simulink model "PMSM_Drive_ForFlight"  (R2025a)
settings: Solver=ode4  StartTime=0.0  StopTime=StopTime  FixedStep=Ts_solver  RelTol=1e-3
values from neighbouring files (symbols this model uses):
  Bm = 1e-3    (= 0.001)    [EMRAX348_DQData.m]    (also in Evolito_D500_DQData.m; pmsm_batt_testbench_data.m)
  C1_pack = (Np/Ns)*c1_cell    [pmsm_batt_testbench_data.m]
  Cap_pack = Np*Cell_Cap    (= 220.5)    [pmsm_batt_testbench_data.m]
  Imax = 1070    [EMRAX348_DQData.m]    (also in Evolito_D500_DQData.m = 1450; pmsm_batt_testbench_data.m = 800)
  Jm_flight = 0.09    [pmsm_batt_testbench_data.m]
  Ki_i = Rs*bw_i    (= 62.8318530718)    [pmsm_batt_testbench_data.m]
  Kp_i = Ld*bw_i    (= 1.25663706144)    [pmsm_batt_testbench_data.m]
  Kt = 1.5*p*psim    (= 3.6)    [pmsm_batt_testbench_data.m]
  Ld = 52e-6    (= 5.2e-05)    [EMRAX348_DQData.m]    (also in Evolito_D500_DQData.m = 4e-05; pmsm_batt_testbench_data.m = 0.0002)
  Lq = 52e-6    (= 5.2e-05)    [EMRAX348_DQData.m]    (also in Evolito_D500_DQData.m = 4e-05; pmsm_batt_testbench_data.m = 0.0002)
  OCV_pack = Ns*ocv_cell    [pmsm_batt_testbench_data.m]
  p = 10    [EMRAX348_DQData.m]    (also in Evolito_D500_DQData.m; pmsm_batt_testbench_data.m = 15)
  psim = 0.06249    [EMRAX348_DQData.m]    (also in Evolito_D500_DQData.m = 0.045; pmsm_batt_testbench_data.m = 0.16)
  R0_pack = (Ns/Np)*rs_cell    [pmsm_batt_testbench_data.m]
  R1_pack = (Ns/Np)*r1_cell    [pmsm_batt_testbench_data.m]
  Rs = 0.00474    [EMRAX348_DQData.m]    (also in Evolito_D500_DQData.m = 0.004; pmsm_batt_testbench_data.m = 0.01)
  SOC0 = 0.90    (= 0.9)    [pmsm_batt_testbench_data.m]
  tau_dc = 1e-4    (= 0.0001)    [pmsm_batt_testbench_data.m]
  trqR_hover = [1500; 1505; 1500; 1505]    [pmsm_batt_testbench_data.m]
undefined symbols (not defined in the file or in its folder): soc_bp
libraries: slpidlib x2, simulink x1
settings Model: Creator=froshoo  LastModifiedBy=wu2408

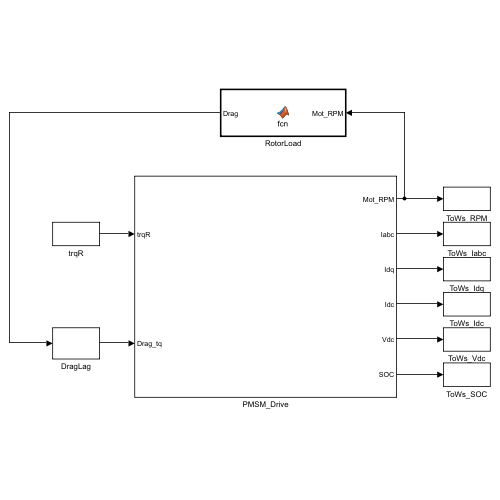
[thumbnail: Simulink's stored preview of the top-level diagram]
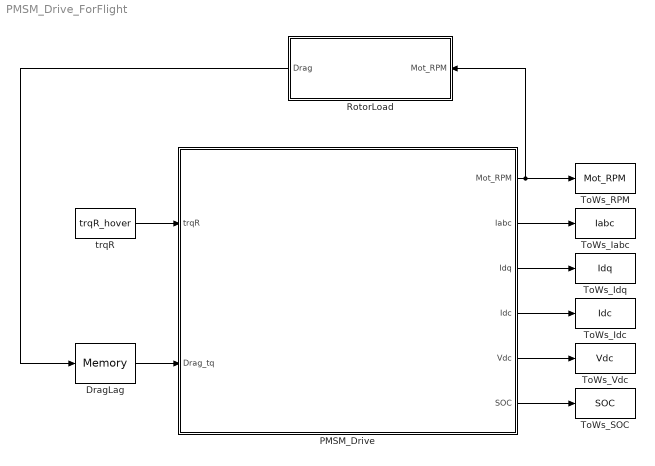
== system PMSM_Drive_ForFlight ==
  DragLag : Memory
  PMSM_Drive : Subsystem
  RotorLoad : MATLAB Function  TreatAsAtomicUnit=on
  ToWs_Iabc : ToWorkspace  VariableName=Iabc  SaveFormat=Timeseries  SampleTime=-1
  ToWs_Idc : ToWorkspace  VariableName=Idc  SaveFormat=Timeseries  SampleTime=-1
  ToWs_Idq : ToWorkspace  VariableName=Idq  SaveFormat=Timeseries  SampleTime=-1
  ToWs_RPM : ToWorkspace  VariableName=Mot_RPM  SaveFormat=Timeseries  SampleTime=-1
  ToWs_SOC : ToWorkspace  VariableName=SOC  SaveFormat=Timeseries  SampleTime=-1
  ToWs_Vdc : ToWorkspace  VariableName=Vdc  SaveFormat=Timeseries  SampleTime=-1
  trqR : Constant  Value=trqR_hover
  wires:
  trqR/1 -> PMSM_Drive/1(trqR)
  RotorLoad/1(Drag) -> DragLag/1
  DragLag/1 -> PMSM_Drive/2(Drag_tq)
  PMSM_Drive/1(Mot_RPM) -> RotorLoad/1(Mot_RPM), ToWs_RPM/1
  PMSM_Drive/2(Iabc) -> ToWs_Iabc/1
  PMSM_Drive/3(Idq) -> ToWs_Idq/1
  PMSM_Drive/4(Idc) -> ToWs_Idc/1
  PMSM_Drive/5(Vdc) -> ToWs_Vdc/1
  PMSM_Drive/6(SOC) -> ToWs_SOC/1

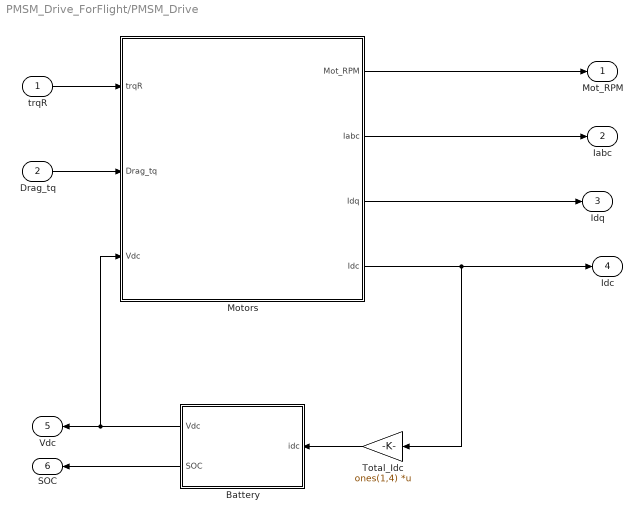
== system PMSM_Drive_ForFlight/PMSM_Drive ==
  trqR : Inport
  Drag_tq : Inport  Port=2
  Battery : Subsystem
  Motors : Subsystem  TreatAsAtomicUnit=on
  Total_Idc : Gain  Gain=ones(1,4)  Multiplication=Matrix(K*u)
  Mot_RPM : Outport
  Iabc : Outport  Port=2
  Idq : Outport  Port=3
  Idc : Outport  Port=4
  Vdc : Outport  Port=5
  SOC : Outport  Port=6
  wires:
  trqR/1 -> Motors/1(trqR)
  Drag_tq/1 -> Motors/2(Drag_tq)
  Battery/1(Vdc) -> Vdc/1, Motors/3(Vdc)
  Motors/1(Mot_RPM) -> Mot_RPM/1
  Motors/2(Iabc) -> Iabc/1
  Motors/3(Idq) -> Idq/1
  Motors/4(Idc) -> Total_Idc/1, Idc/1
  Total_Idc/1 -> Battery/1(idc)
  Battery/2(SOC) -> SOC/1

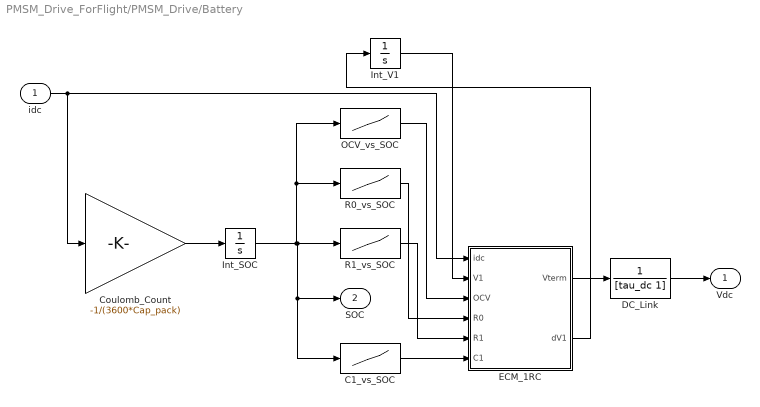
== system PMSM_Drive_ForFlight/PMSM_Drive/Battery ==
  idc : Inport
  C1_vs_SOC : Lookup_n-D  NumberOfTableDimensions=1  BreakpointsForDimension1=soc_bp  Table=C1_pack  InternalRulePriority=Speed  RndMeth=Simplest
  Coulomb_Count : Gain  Gain=-1/(3600*Cap_pack)
  DC_Link : TransferFcn  Denominator=[tau_dc 1]
  ECM_1RC : MATLAB Function  TreatAsAtomicUnit=on
  Int_SOC : Integrator  InitialCondition=SOC0
  Int_V1 : Integrator
  OCV_vs_SOC : Lookup_n-D  NumberOfTableDimensions=1  BreakpointsForDimension1=soc_bp  Table=OCV_pack  InternalRulePriority=Speed  RndMeth=Simplest
  R0_vs_SOC : Lookup_n-D  NumberOfTableDimensions=1  BreakpointsForDimension1=soc_bp  Table=R0_pack  InternalRulePriority=Speed  RndMeth=Simplest
  R1_vs_SOC : Lookup_n-D  NumberOfTableDimensions=1  BreakpointsForDimension1=soc_bp  Table=R1_pack  InternalRulePriority=Speed  RndMeth=Simplest
  Vdc : Outport
  SOC : Outport  Port=2
  wires:
  Int_V1/1 -> ECM_1RC/2(V1)
  idc/1 -> ECM_1RC/1(idc), Coulomb_Count/1
  Coulomb_Count/1 -> Int_SOC/1
  R0_vs_SOC/1 -> ECM_1RC/4(R0)
  Int_SOC/1 -> C1_vs_SOC/1, SOC/1, R1_vs_SOC/1, OCV_vs_SOC/1, R0_vs_SOC/1
  OCV_vs_SOC/1 -> ECM_1RC/3(OCV)
  R1_vs_SOC/1 -> ECM_1RC/5(R1)
  C1_vs_SOC/1 -> ECM_1RC/6(C1)
  ECM_1RC/1(Vterm) -> DC_Link/1
  ECM_1RC/2(dV1) -> Int_V1/1
  DC_Link/1 -> Vdc/1

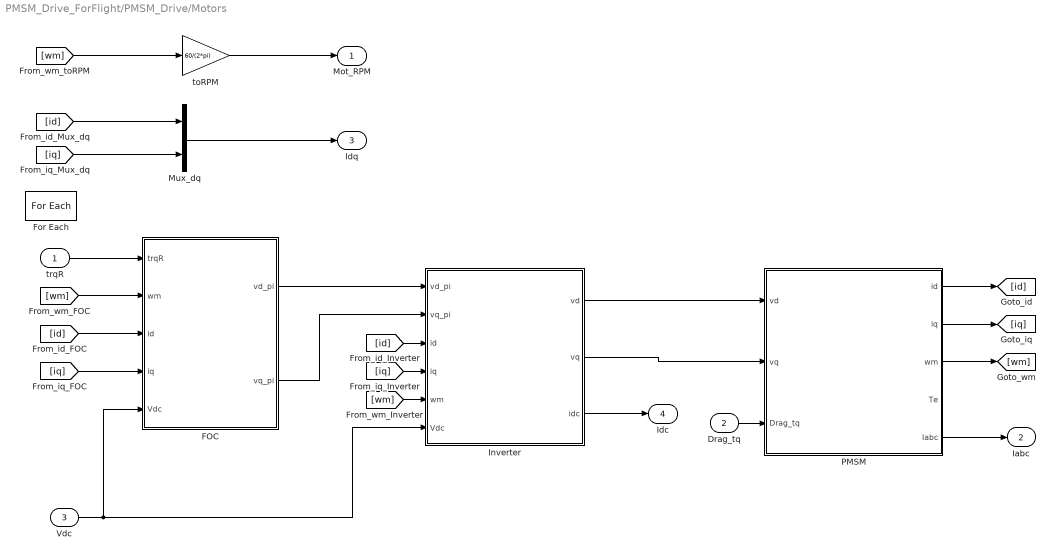
== system PMSM_Drive_ForFlight/PMSM_Drive/Motors ==
  trqR : Inport  Partition=on  PartitionDimension=1  PartitionWidth=1  PartitionOffset=0
  Drag_tq : Inport  Port=2  Partition=on  PartitionDimension=1  PartitionWidth=1  PartitionOffset=0
  Vdc : Inport  Port=3
  FOC : Subsystem
  For Each : ForEach  DisableCoverage=on  SpecifiedNumIters=4
  Inverter : Subsystem
  Mux_dq : Mux  Inputs=2
  PMSM : Subsystem
  toRPM : Gain  Gain=60/(2*pi)
  Mot_RPM : Outport  ConcatenationDimension=1
  Iabc : Outport  Port=2  ConcatenationDimension=1
  Idq : Outport  Port=3  ConcatenationDimension=1
  Idc : Outport  Port=4  ConcatenationDimension=1
  wires:
  [wm] -> Inverter/5(wm)
  [wm] -> toRPM/1
  [iq] -> Mux_dq/2
  [wm] -> FOC/2(wm)
  PMSM/5(Iabc) -> Iabc/1
  PMSM/3(wm) -> [wm]
  [id] -> Mux_dq/1
  trqR/1 -> FOC/1(trqR)
  [id] -> FOC/3(id)
  [iq] -> Inverter/4(iq)
  [iq] -> FOC/4(iq)
  Vdc/1 -> Inverter/6(Vdc), FOC/5(Vdc)
  toRPM/1 -> Mot_RPM/1
  Mux_dq/1 -> Idq/1
  FOC/2(vq_pi) -> Inverter/2(vq_pi)
  FOC/1(vd_pi) -> Inverter/1(vd_pi)
  [id] -> Inverter/3(id)
  Inverter/3(idc) -> Idc/1
  Inverter/2(vq) -> PMSM/2(vq)
  Inverter/1(vd) -> PMSM/1(vd)
  Drag_tq/1 -> PMSM/3(Drag_tq)
  PMSM/2(iq) -> [iq]
  PMSM/1(id) -> [id]

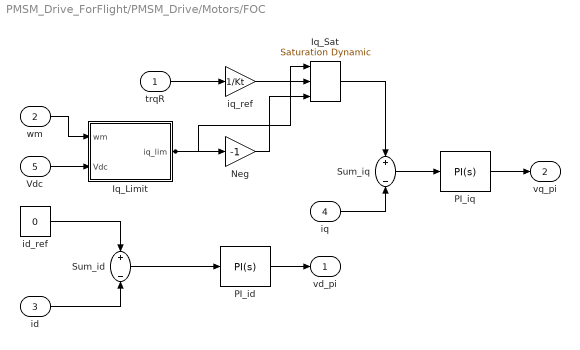
== system PMSM_Drive_ForFlight/PMSM_Drive/Motors/FOC ==
  trqR : Inport
  wm : Inport  Port=2
  id : Inport  Port=3
  iq : Inport  Port=4
  Vdc : Inport  Port=5
  Iq_Limit : MATLAB Function  TreatAsAtomicUnit=on
  Iq_Sat : simulink/Discontinuities/Saturation Dynamic  OutMin=[]  OutMax=[]  OutDataTypeStr=Inherit: Same as second input  OutDataType=fixdt(1, 16)  OutScaling=2^-10  DoSatur=off
  Neg : Gain  Gain=-1
  PI_id : slpidlib/PID Controller  Controller=PI  Form=Parallel  TimeDomain=Continuous-time  UseExternalTs=off  SampleTime=-1  IntegratorMethod=Forward Euler  FilterMethod=Forward Euler  ControllerParametersSource=internal  P=Kp_i  I=Ki_i  UseKiTs=off  D=0  UseExternalDerivativeSource=off  N=100  UseFilter=on  TunerSelectOption=Transfer Function Based (PID Tuner App)  InitialConditionSource=internal  InitialConditionForIntegrator=0  InitialConditionForFilter=0  DifferentiatorICPrevScaledInput=0  ExternalReset=none  TrackingMode=off  Kt=1  LimitOutput=off  SatLimitsSource=internal  UpperSaturationLimit=inf  LowerSaturationLimit=-inf  LinearizeAsGain=on  AntiWindupMode=none  Kb=1  LimitIntegrator=off  UpperIntegratorSaturationLimit=inf  LowerIntegratorSaturationLimit=-inf  POutMin=[]  POutMax=[]  IOutMin=[]  IOutMax=[]  DOutMin=[]  DOutMax=[]  NOutMin=[]  NOutMax=[]  SumOutMin=[]  SumOutMax=[]  SaturationOutMin=[]  SaturationOutMax=[]  PParamMin=[]  PParamMax=[]  IParamMin=[]  IParamMax=[]  DParamMin=[]  DParamMax=[]  NParamMin=[]  NParamMax=[]  KbParamMin=[]  KbParamMax=[]  KtParamMin=[]  KtParamMax=[]  KbOutMin=[]  KbOutMax=[]  KtOutMin=[]  KtOutMax=[]  IntegratorOutMin=[]  IntegratorOutMax=[]  FilterOutMin=[]  FilterOutMax=[]  SumI1OutMin=[]  SumI1OutMax=[]  SumI2OutMin=[]  SumI2OutMax=[]  SumI3OutMin=[]  SumI3OutMax=[]  SumI4OutMin=[]  SumI4OutMax=[]  SumDOutMin=[]  SumDOutMax=[]  DifferentiatorOutMin=[]  DifferentiatorOutMax=[]  FilterDiffOutCoefMin=[]  FilterDiffOutCoefMax=[]  ReciprocalOutMin=[]  ReciprocalOutMax=[]  SumDenOutMin=[]  SumDenOutMax=[]  SumNumOutMin=[]  SumNumOutMax=[]  DivideOutMin=[]  DivideOutMax=[]  UdiffTsProdOutMin=[]  UdiffTsProdOutMax=[]  NTsProdOutMin=[]  NTsProdOutMax=[]  UintegralTsProdOutMin=[]  UintegralTsProdOutMax=[]  UngainTsProdOutMin=[]  UngainTsProdOutMax=[]  ClampingZeroOutDataTypeStr=Inherit: Inherit via back propagation  ClampingZeroOutMin=[]  ClampingZeroOutMax=[]  FilterDenConstantOutDataTypeStr=Inherit: Inherit via back propagation  FilterDenConstantOutMin=[]  FilterDenConstantOutMax=[]  PCopyOutDataTypeStr=Inherit: Inherit via back propagation  PCopyOutMin=[]  PCopyOutMax=[]  NCopyOutDataTypeStr=Inherit: Inherit via back propagation  NCopyOutMin=[]  NCopyOutMax=[]  IntegratorContinuousStateAttributes=''  IntegratorStateMustResolveToSignalObject=off  IntegratorRTWStateStorageClass=Auto  FilterContinuousStateAttributes=''  FilterStateMustResolveToSignalObject=off  FilterRTWStateStorageClass=Auto  ParallelPVariant=InternalParameters  IdealPVariant=Disabled  IVariant=InternalParameters  DVariant=Disabled  IntegratorVariant=Continuous  SatVariant=Disabled  AWVariant=Passthrough  PCopyVariant=Disabled  TRVariant=Disabled  FdbkBlocksVariant=Forward  IdealPFdbkVariant=Disabled  SatFdbkVariant=Disabled  DerivativeFilterVariant=Disabled  NVariant=Disabled  NCopyVariant=Disabled_SignalSpec  FilterICVariant=Disabled  IntegratorICVariant=InternalICs  ExternalResetVariant=Disabled  TRSumVariant=Passthrough  SumFdbkVariant=Disabled  SumVariant=Sum_PI  TsampFilterVariant=InternalTs  TsampNgainVariant=Passthrough  TsampIntegralVariant=Disabled_SignalSpec  ExternalSaturationOutDataTypeStr=Inherit: Same as second input  DerivativeSourceVariant=Disabled  PreIntVariant=InternalPreInt
  PI_iq : slpidlib/PID Controller  Controller=PI  Form=Parallel  TimeDomain=Continuous-time  UseExternalTs=off  SampleTime=-1  IntegratorMethod=Forward Euler  FilterMethod=Forward Euler  ControllerParametersSource=internal  P=Kp_i  I=Ki_i  UseKiTs=off  D=0  UseExternalDerivativeSource=off  N=100  UseFilter=on  TunerSelectOption=Transfer Function Based (PID Tuner App)  InitialConditionSource=internal  InitialConditionForIntegrator=0  InitialConditionForFilter=0  DifferentiatorICPrevScaledInput=0  ExternalReset=none  TrackingMode=off  Kt=1  LimitOutput=off  SatLimitsSource=internal  UpperSaturationLimit=inf  LowerSaturationLimit=-inf  LinearizeAsGain=on  AntiWindupMode=none  Kb=1  LimitIntegrator=off  UpperIntegratorSaturationLimit=inf  LowerIntegratorSaturationLimit=-inf  POutMin=[]  POutMax=[]  IOutMin=[]  IOutMax=[]  DOutMin=[]  DOutMax=[]  NOutMin=[]  NOutMax=[]  SumOutMin=[]  SumOutMax=[]  SaturationOutMin=[]  SaturationOutMax=[]  PParamMin=[]  PParamMax=[]  IParamMin=[]  IParamMax=[]  DParamMin=[]  DParamMax=[]  NParamMin=[]  NParamMax=[]  KbParamMin=[]  KbParamMax=[]  KtParamMin=[]  KtParamMax=[]  KbOutMin=[]  KbOutMax=[]  KtOutMin=[]  KtOutMax=[]  IntegratorOutMin=[]  IntegratorOutMax=[]  FilterOutMin=[]  FilterOutMax=[]  SumI1OutMin=[]  SumI1OutMax=[]  SumI2OutMin=[]  SumI2OutMax=[]  SumI3OutMin=[]  SumI3OutMax=[]  SumI4OutMin=[]  SumI4OutMax=[]  SumDOutMin=[]  SumDOutMax=[]  DifferentiatorOutMin=[]  DifferentiatorOutMax=[]  FilterDiffOutCoefMin=[]  FilterDiffOutCoefMax=[]  ReciprocalOutMin=[]  ReciprocalOutMax=[]  SumDenOutMin=[]  SumDenOutMax=[]  SumNumOutMin=[]  SumNumOutMax=[]  DivideOutMin=[]  DivideOutMax=[]  UdiffTsProdOutMin=[]  UdiffTsProdOutMax=[]  NTsProdOutMin=[]  NTsProdOutMax=[]  UintegralTsProdOutMin=[]  UintegralTsProdOutMax=[]  UngainTsProdOutMin=[]  UngainTsProdOutMax=[]  ClampingZeroOutDataTypeStr=Inherit: Inherit via back propagation  ClampingZeroOutMin=[]  ClampingZeroOutMax=[]  FilterDenConstantOutDataTypeStr=Inherit: Inherit via back propagation  FilterDenConstantOutMin=[]  FilterDenConstantOutMax=[]  PCopyOutDataTypeStr=Inherit: Inherit via back propagation  PCopyOutMin=[]  PCopyOutMax=[]  NCopyOutDataTypeStr=Inherit: Inherit via back propagation  NCopyOutMin=[]  NCopyOutMax=[]  IntegratorContinuousStateAttributes=''  IntegratorStateMustResolveToSignalObject=off  IntegratorRTWStateStorageClass=Auto  FilterContinuousStateAttributes=''  FilterStateMustResolveToSignalObject=off  FilterRTWStateStorageClass=Auto  ParallelPVariant=InternalParameters  IdealPVariant=Disabled  IVariant=InternalParameters  DVariant=Disabled  IntegratorVariant=Continuous  SatVariant=Disabled  AWVariant=Passthrough  PCopyVariant=Disabled  TRVariant=Disabled  FdbkBlocksVariant=Forward  IdealPFdbkVariant=Disabled  SatFdbkVariant=Disabled  DerivativeFilterVariant=Disabled  NVariant=Disabled  NCopyVariant=Disabled_SignalSpec  FilterICVariant=Disabled  IntegratorICVariant=InternalICs  ExternalResetVariant=Disabled  TRSumVariant=Passthrough  SumFdbkVariant=Disabled  SumVariant=Sum_PI  TsampFilterVariant=InternalTs  TsampNgainVariant=Passthrough  TsampIntegralVariant=Disabled_SignalSpec  ExternalSaturationOutDataTypeStr=Inherit: Same as second input  DerivativeSourceVariant=Disabled  PreIntVariant=InternalPreInt
  Sum_id : Sum  Inputs=+-
  Sum_iq : Sum  Inputs=+-
  id_ref : Constant  Value=0
  iq_ref : Gain  Gain=1/Kt
  vd_pi : Outport
  vq_pi : Outport  Port=2
  wires:
  trqR/1 -> iq_ref/1
  id/1 -> Sum_id/2
  wm/1 -> Iq_Limit/1(wm)
  iq_ref/1 -> Iq_Sat/2
  Vdc/1 -> Iq_Limit/2(Vdc)
  Sum_iq/1 -> PI_iq/1
  id_ref/1 -> Sum_id/1
  Sum_id/1 -> PI_id/1
  Iq_Limit/1(iq_lim) -> Iq_Sat/1, Neg/1
  Neg/1 -> Iq_Sat/3
  PI_id/1 -> vd_pi/1
  Iq_Sat/1 -> Sum_iq/1
  iq/1 -> Sum_iq/2
  PI_iq/1 -> vq_pi/1

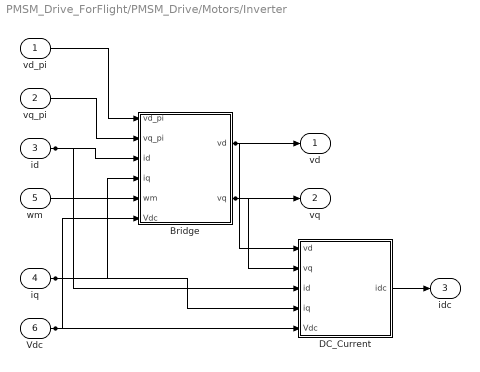
== system PMSM_Drive_ForFlight/PMSM_Drive/Motors/Inverter ==
  vd_pi : Inport
  vq_pi : Inport  Port=2
  id : Inport  Port=3
  iq : Inport  Port=4
  wm : Inport  Port=5
  Vdc : Inport  Port=6
  Bridge : MATLAB Function  TreatAsAtomicUnit=on
  DC_Current : MATLAB Function  TreatAsAtomicUnit=on
  vd : Outport
  vq : Outport  Port=2
  idc : Outport  Port=3
  wires:
  Bridge/1(vd) -> vd/1, DC_Current/1(vd)
  vd_pi/1 -> Bridge/1(vd_pi)
  iq/1 -> DC_Current/4(iq), Bridge/4(iq)
  vq_pi/1 -> Bridge/2(vq_pi)
  Vdc/1 -> DC_Current/5(Vdc), Bridge/6(Vdc)
  id/1 -> DC_Current/3(id), Bridge/3(id)
  wm/1 -> Bridge/5(wm)
  Bridge/2(vq) -> vq/1, DC_Current/2(vq)
  DC_Current/1(idc) -> idc/1

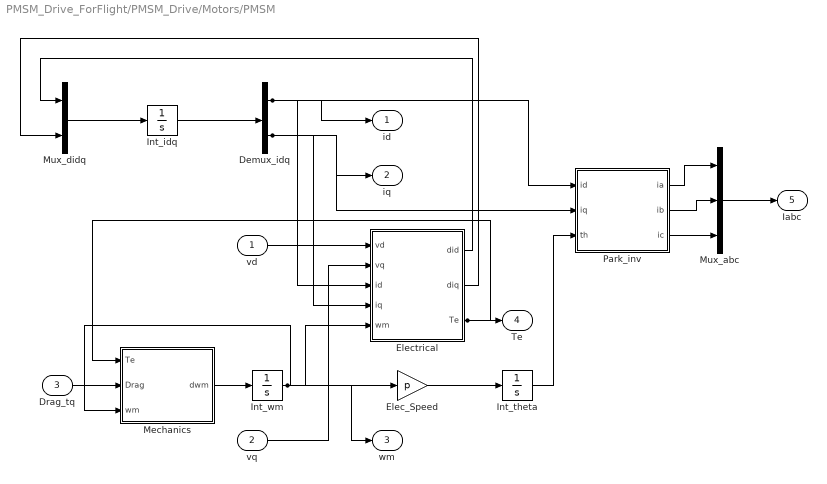
== system PMSM_Drive_ForFlight/PMSM_Drive/Motors/PMSM ==
  vd : Inport
  vq : Inport  Port=2
  Drag_tq : Inport  Port=3
  Demux_idq : Demux  Outputs=2
  Elec_Speed : Gain  Gain=p
  Electrical : MATLAB Function  TreatAsAtomicUnit=on
  Int_idq : Integrator  InitialCondition=[0;0]
  Int_theta : Integrator
  Int_wm : Integrator
  Mechanics : MATLAB Function  TreatAsAtomicUnit=on
  Mux_abc : Mux  Inputs=3
  Mux_didq : Mux  Inputs=2
  Park_inv : MATLAB Function  TreatAsAtomicUnit=on
  id : Outport
  iq : Outport  Port=2
  wm : Outport  Port=3
  Te : Outport  Port=4
  Iabc : Outport  Port=5
  wires:
  Mux_didq/1 -> Int_idq/1
  Demux_idq/2 -> Park_inv/2(iq), Electrical/4(iq), iq/1
  Mechanics/1(dwm) -> Int_wm/1
  Drag_tq/1 -> Mechanics/2(Drag)
  Int_wm/1 -> Electrical/5(wm), wm/1, Mechanics/3(wm), Elec_Speed/1
  vd/1 -> Electrical/1(vd)
  Int_idq/1 -> Demux_idq/1
  Demux_idq/1 -> id/1, Electrical/3(id), Park_inv/1(id)
  vq/1 -> Electrical/2(vq)
  Electrical/1(did) -> Mux_didq/1
  Electrical/2(diq) -> Mux_didq/2
  Electrical/3(Te) -> Mechanics/1(Te), Te/1
  Elec_Speed/1 -> Int_theta/1
  Int_theta/1 -> Park_inv/3(th)
  Park_inv/1(ia) -> Mux_abc/1
  Park_inv/2(ib) -> Mux_abc/2
  Park_inv/3(ic) -> Mux_abc/3
  Mux_abc/1 -> Iabc/1

== matlab function PMSM_Drive_ForFlight/RotorLoad ==
  data: Mot_RPM input size=4; Drag output size=4; k_drag parameter
function Drag = fcn(Mot_RPM, k_drag)
wm   = Mot_RPM*2*pi/60;
Drag = k_drag .* wm .* abs(wm);

== matlab function PMSM_Drive_ForFlight/PMSM_Drive/Motors/Inverter/Bridge ==
  data: vd_pi input size=1; vd output size=1; vq_pi input size=1; id input size=1; iq input size=1; wm input size=1; Vdc input size=1; vq output size=1; p parameter; Ld parameter; Lq parameter; psim parameter
function [vd, vq] = fcn(vd_pi, vq_pi, id, iq, wm, Vdc, p, Ld, Lq, psim)
we   = p*wm;
vd_c = vd_pi - we*Lq*iq;
vq_c = vq_pi + we*(Ld*id + psim);
Vmax = Vdc/sqrt(3);
vd      = max(-Vmax, min(Vmax, vd_c));
vq_room = sqrt(max(Vmax^2 - vd^2, 0));
vq      = max(-vq_room, min(vq_room, vq_c));

== matlab function PMSM_Drive_ForFlight/PMSM_Drive/Motors/FOC/Iq_Limit ==
  data: wm input size=1; iq_lim output size=1; Vdc input size=1; p parameter; psim parameter; Lq parameter; Imax parameter
function iq_lim = fcn(wm, Vdc, p, psim, Lq, Imax)
we   = p*abs(wm);
Vmax = Vdc/sqrt(3);
Eb   = we*psim;
marg = Vmax^2 - Eb^2;
if we < 1 || marg <= 0
    iq_v = Imax;
else
    iq_v = sqrt(marg)/(we*Lq);
end
iq_lim = min(Imax, iq_v);

== matlab function PMSM_Drive_ForFlight/PMSM_Drive/Motors/Inverter/DC_Current ==
  data: vd input size=1; idc output size=1; vq input size=1; id input size=1; iq input size=1; Vdc input size=1
function idc = fcn(vd, vq, id, iq, Vdc)
Pac = 1.5*(vd*id + vq*iq);
idc = Pac/max(Vdc, 1);

== matlab function PMSM_Drive_ForFlight/PMSM_Drive/Motors/PMSM/Electrical ==
  data: vd input size=1; did output size=1; vq input size=1; id input size=1; iq input size=1; wm input size=1; diq output size=1; Te output size=1; p parameter; Rs parameter; Ld parameter; Lq parameter; psim parameter
function [did, diq, Te] = fcn(vd, vq, id, iq, wm, p, Rs, Ld, Lq, psim)
we  = p*wm;
did = (vd - Rs*id + we*Lq*iq)/Ld;
diq = (vq - Rs*iq - we*(Ld*id + psim))/Lq;
Te  = 1.5*p*(psim*iq + (Ld - Lq)*id*iq);

== matlab function PMSM_Drive_ForFlight/PMSM_Drive/Motors/PMSM/Mechanics ==
  data: Te input size=1; dwm output size=1; Drag input size=1; wm input size=1; Bm parameter; Jm_flight parameter
function dwm = fcn(Te, Drag, wm, Bm, Jm_flight)
dwm = (Te - Drag - Bm*wm)/Jm_flight;

== matlab function PMSM_Drive_ForFlight/PMSM_Drive/Motors/PMSM/Park_inv ==
  data: id input size=1; ia output size=1; iq input size=1; th input size=1; ib output size=1; ic output size=1
function [ia, ib, ic] = fcn(id, iq, th)
ia = id*cos(th)        - iq*sin(th);
ib = id*cos(th-2*pi/3) - iq*sin(th-2*pi/3);
ic = id*cos(th+2*pi/3) - iq*sin(th+2*pi/3);

== matlab function PMSM_Drive_ForFlight/PMSM_Drive/Battery/ECM_1RC ==
  data: idc input size=1; Vterm output size=1; V1 input size=1; OCV input size=1; R0 input size=1; R1 input size=1; C1 input size=1; dV1 output size=1
function [Vterm, dV1] = fcn(idc, V1, OCV, R0, R1, C1)
Vterm = OCV - idc*R0 - V1;
dV1   = idc/C1 - V1/(R1*C1);
